simulink model "model4"  (R2021a)
settings: Solver=VariableStepAuto  StartTime=0.0  StopTime=10.0  MaxStep=1e-4  RelTol=1e-3
undefined symbols (not defined in the file): D, K1, K2, m1, m2, sys_d
settings Model: Creator=Luka  LastModifiedBy=Luka

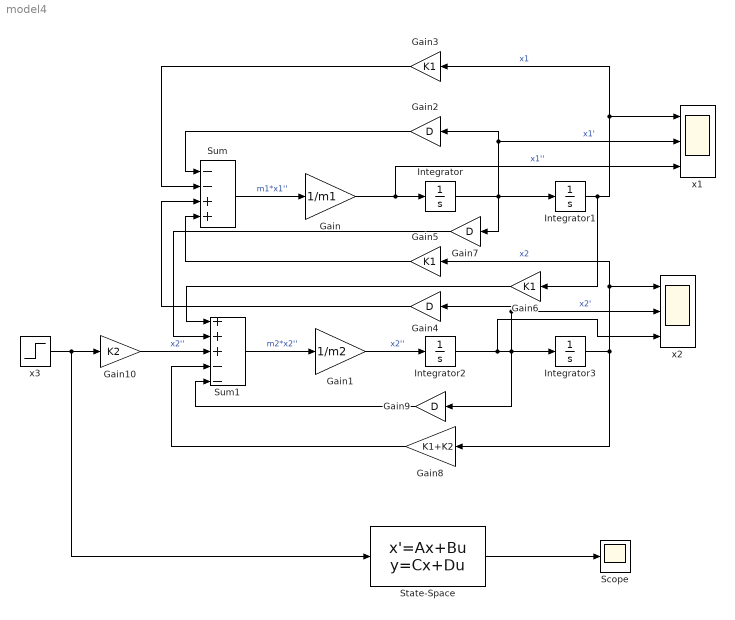
== system model4 ==
  Gain : Gain  Gain=1/m1
  Gain1 : Gain  Gain=1/m2
  Gain10 : Gain  Gain=K2
  Gain{2,4,7,9} (4 alike) : Gain  Gain=D
  Gain3 : Gain  Gain=K1
  Gain5 : Gain  Gain=K1
  Gain6 : Gain  Gain=K1
  Gain8 : Gain  Gain=K1+K2
  Integrator{,1..3} (4 alike) : Integrator
  Scope : Scope
  State-Space : StateSpace  A=sys_d.A  B=sys_d.B  C=[sys_d.C; eye(4)]  D=[sys_d.D; zeros(4,1)]  InitialCondition=0
  Sum : Sum  Inputs=--++
  Sum1 : Sum  Inputs=+++--
  x1 : Scope  NumInputPorts=3
  x2 : Scope  NumInputPorts=3
  x3 : Step  Time=0  SampleTime=0
  wires:
  Integrator/1 -> Gain7/1, Gain2/1, x1/2, Integrator1/1  "x1'"
  Integrator2/1 -> x2/3, Gain4/1, x2/2, Gain9/1, Integrator3/1  "x2'"
  Integrator1/1 -> Gain3/1, x1/1, Gain6/1  "x1"
  Integrator3/1 -> Gain8/1, x2/1, Gain5/1  "x2"
  Gain/1 -> x1/3, Integrator/1  "x1''"
  Sum/1 -> Gain/1  "m1*x1''"
  Sum1/1 -> Gain1/1  "m2*x2''"
  Gain1/1 -> Integrator2/1  "x2''"
  Gain2/1 -> Sum/1
  Gain3/1 -> Sum/2
  Gain5/1 -> Sum/4
  Gain4/1 -> Sum/3
  Gain6/1 -> Sum1/1
  Gain7/1 -> Sum1/2
  Gain9/1 -> Sum1/5
  Gain8/1 -> Sum1/4
  Gain10/1 -> Sum1/3  "x2''"
  x3/1 -> State-Space/1, Gain10/1
  State-Space/1 -> Scope/1
